simulink model "trajectories"  (R2016b)
settings: Solver=FixedStepAuto  StartTime=0.0  StopTime=20  FixedStep=.1  RelTol=1e-3
undefined symbols (not defined in the file or in its folder): sigbuilder_block
libraries: simulink x3, powerlib_meascontrol x1
settings Model: Creator=Kamran  LastModifiedBy=Kamran

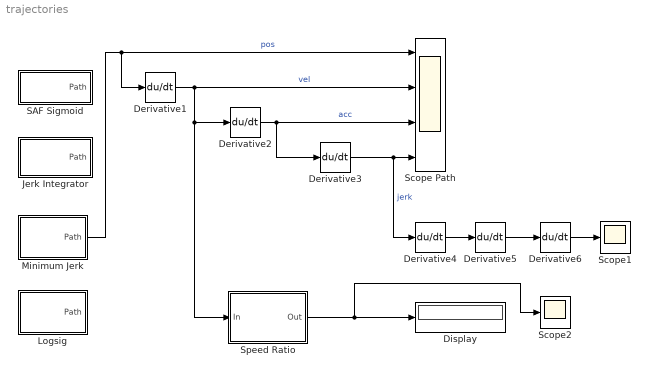
== system trajectories ==
  Derivative{1..6} (6 alike) : Derivative
  Display : Display
  Jerk Integrator : Subsystem
  Logsig : Subsystem
  Minimum Jerk : Subsystem  mask{xi=0, xf=3, d=10, start=5}
      mask prompts: xi "Initial Position"; xf "Final Position"; d "Duration"; start "Start Time"
      mask help: Neville Hogan (1984a) noted that smoothness can be quantified as a function of jerk. This function, among all possible functions, has the minimum jerk cost. Which means that some function that happens to have its sixth derivative equal to zero will minimize your jerk function.
      mask Help: http://www.shadmehrlab.org/book/minimum_jerk/minimumjerk.htm
  SAF Sigmoid : Subsystem
  Scope Path : Scope  NumInputPorts=4
  Scope1 : Scope
  Scope2 : Scope
  Speed Ratio : Subsystem  mask{ts=5, tf=15}
      mask prompts: ts "Measure Start Time"; tf "Measure End Time"
      mask help: Ratio of peak speed to average speed (r). Psychophysical experiments reveal that your reaching movements have a ratio r = 1.75.
      mask Help: http://www.shadmehrlab.org/book/minimum_jerk/minimumjerk.htm
  wires:
  Minimum Jerk/1(Path) -> Scope Path/1, Derivative1/1  "pos"
  Derivative1/1 -> Derivative2/1, Speed Ratio/1(In), Scope Path/2  "vel"
  Derivative3/1 -> Scope Path/4, Derivative4/1  "jerk"
  Derivative2/1 -> Derivative3/1, Scope Path/3  "acc"
  Speed Ratio/1(Out) -> Scope2/1, Display/1
  Derivative5/1 -> Derivative6/1
  Derivative4/1 -> Derivative5/1
  Derivative6/1 -> Scope1/1

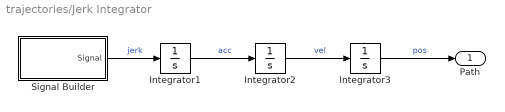
== system trajectories/Jerk Integrator ==
  Integrator1 : Integrator
  Integrator2 : Integrator
  Integrator3 : Integrator
  Signal Builder : Subsystem  Tag=STV Subsys  LoadFcn=sigbuilder_block('load');  StartFcn=sigbuilder_block('start');  StopFcn=sigbuilder_block('stop');  ClipboardFcn=sigbuilder_block('clipboard');  mask(Sigbuilder block){tuvar=[0:10]}
      mask help: Simulink:masks:SigbuilderBlock_MD
      mask init:
      | if ~strcmp(get_param(bdroot(gcbh),'SimulationStatus'),'stopped') tuvar = sigbuilder_block('maskInit'); end
      settings: CopyFcn=sigbuilder_block('copy');  DeleteFcn=sigbuilder_block('delete');  ModelCloseFcn=sigbuilder_block('modelClose');  PreSaveFcn=sigbuilder_block('preSave');  PauseFcn=sigbuilder_block('pause');  ContinueFcn=sigbuilder_block('continue');  NameChangeFcn=sigbuilder_block('namechange');  OpenFcn=sigbuilder_block('open',[6 30 1188 546.75 ]);  CloseFcn=sigbuilder_block('close');
      mask Display: plot(0, 0, 100, 100,[2, 2, 32, 32, 2], [68, 8, 8, 68, 68],[32, 2], [38, 38], [32, 19, 2],[53, 60, 44], [32, 17, 17, 2],[16, 16, 31, 31]);txt = getActiveGroup(gcbh);text(2, 100, txt,'verticalAlignment', 'top');
  Path : Outport
  wires:
  Integrator1/1 -> Integrator2/1  "acc"
  Integrator2/1 -> Integrator3/1  "vel"
  Signal Builder/1(Signal) -> Integrator1/1  "jerk"
  Integrator3/1 -> Path/1  "pos"

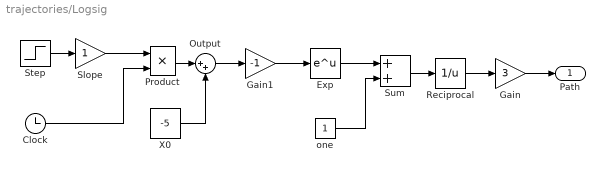
== system trajectories/Logsig ==
  Clock : Clock
      settings: DisableCoverage=on
  Exp : Math  SaturateOnIntegerOverflow=on
  Gain : Gain  Gain=3
  Gain1 : Gain  Gain=-1  SaturateOnIntegerOverflow=on  OutDataTypeStr=Inherit: Same as input  ParamDataTypeStr=Inherit: Same as input
  Output : Sum  Inputs=|++  SaturateOnIntegerOverflow=on  InputSameDT=on  OutDataTypeStr=Inherit: Same as first input
  Product : Product  DisableCoverage=on  SaturateOnIntegerOverflow=on  InputSameDT=on  OutDataTypeStr=Inherit: Same as first input
  Reciprocal : Math  Operator=reciprocal  SaturateOnIntegerOverflow=on
  Slope : Gain
  Step : Step  DisableCoverage=on  Time=0  SampleTime=0
  Sum : Sum  SaturateOnIntegerOverflow=on  InputSameDT=on  OutDataTypeStr=Inherit: Same as first input
  X0 : Constant  Value=-5
  one : Constant
  Path : Outport
  wires:
  Slope/1 -> Product/1
  Step/1 -> Slope/1
  Product/1 -> Output/1
  X0/1 -> Output/2
  Clock/1 -> Product/2
  Sum/1 -> Reciprocal/1
  one/1 -> Sum/2
  Exp/1 -> Sum/1
  Gain1/1 -> Exp/1
  Output/1 -> Gain1/1
  Gain/1 -> Path/1
  Reciprocal/1 -> Gain/1

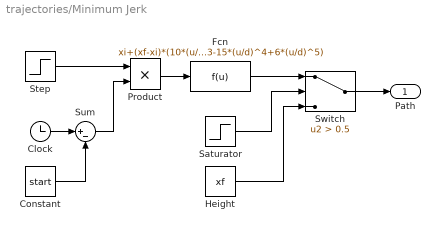
== system trajectories/Minimum Jerk ==
  Clock : Clock
  Constant : Constant  Value=start
  Fcn : Fcn  Expr=xi+(xf-xi)*(10*(u/d)^3-15*(u/d)^4+6*(u/d)^5)
  Height : Constant  Value=xf
  Product : Product
  Saturator : Step  Time=start+d  Before=1  After=0  SampleTime=0
  Step : Step  Time=start  SampleTime=0
  Sum : Sum  Inputs=|+-
  Switch : Switch  Criteria=u2 > Threshold  Threshold=0.5
  Path : Outport
  wires:
  Product/1 -> Fcn/1
  Fcn/1 -> Switch/1
  Step/1 -> Product/1
  Clock/1 -> Sum/1
  Constant/1 -> Sum/2
  Sum/1 -> Product/2
  Saturator/1 -> Switch/2
  Height/1 -> Switch/3
  Switch/1 -> Path/1

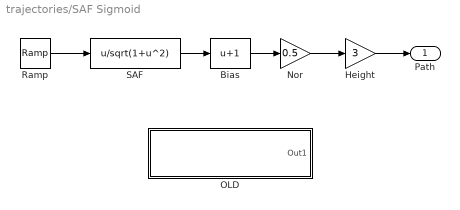
== system trajectories/SAF Sigmoid ==
  Bias : Bias  Bias=1
  Height : Gain  Gain=3
  Nor : Gain  Gain=0.5
  OLD : Subsystem
  Ramp : simulink/Sources/Ramp  slope=1  start=0  X0=-5
  SAF : Fcn  Expr=u/sqrt(1+u^2)
  Path : Outport
  wires:
  Ramp/1 -> SAF/1
  SAF/1 -> Bias/1
  Height/1 -> Path/1
  Bias/1 -> Nor/1
  Nor/1 -> Height/1

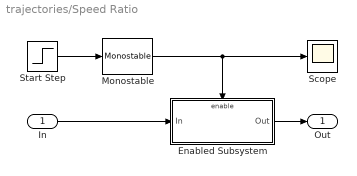
== system trajectories/Speed Ratio ==
  In : Inport
  Enabled Subsystem : Subsystem  TreatAsAtomicUnit=on
  Monostable : powerlib_meascontrol/Logic/Monostable  EdgeDetect=Rising  PulseDuration=tf-ts  ic=0  Ts=0
  Scope : Scope
  Start Step : Step  Time=ts  SampleTime=0
  Out : Outport
  wires:
  In/1 -> Enabled Subsystem/1(In)
  Enabled Subsystem/1(Out) -> Out/1
  Start Step/1 -> Monostable/1
  Monostable/1 -> Scope/1, Enabled Subsystem/Enable

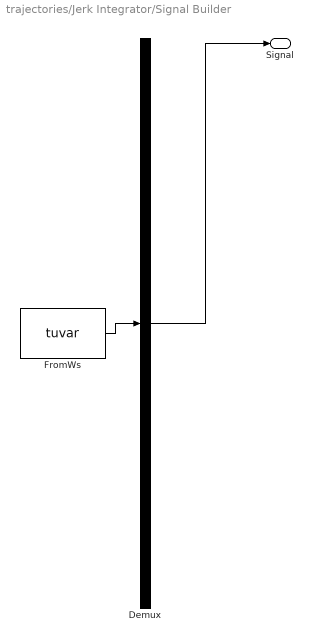
== system trajectories/Jerk Integrator/Signal Builder ==
  Demux : Demux  Tag=STV Demux  Outputs=1
  FromWs : FromWorkspace  Tag=STV FromWs  VariableName=tuvar  SampleTime=0
      SigBuilderData=|
      | common.afterFinalStr = 'Extrapolate'
      | common.sampleTime = 0
      | dataSet.timeRange = [0 10]
      | dataSet.name = 'Group'
      | sbobj.Groups.Name = 'Group'
      | sbobj.Groups.Signals.Name = 'Signal'
      | sbobj.Groups.Signals.XData = [0 1 1 2 2 3 3 4 4 5 5 10]
      | sbobj.Groups.Signals.YData = [1 1 -1 -1 0 0 -1 -1 1 1 0 0]
  Signal : Outport  Tag=STV Outport
  wires:
  Demux/1 -> Signal/1
  FromWs/1 -> Demux/1

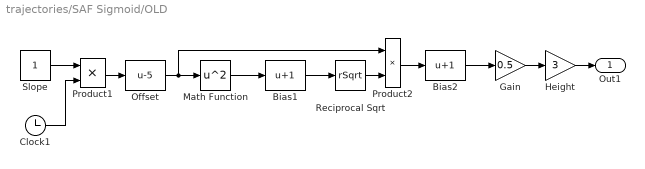
== system trajectories/SAF Sigmoid/OLD ==
  Bias1 : Bias  Bias=1
  Bias2 : Bias  Bias=1
  Clock1 : Clock
      settings: DisableCoverage=on
  Gain : Gain  Gain=0.5
  Height : Gain  Gain=3
  Math Function : Math  Operator=square  SaturateOnIntegerOverflow=on
  Offset : Bias  Bias=-5
  Product1 : Product  DisableCoverage=on  SaturateOnIntegerOverflow=on  InputSameDT=on  OutDataTypeStr=Inherit: Same as first input
  Product2 : Product  DisableCoverage=on  SaturateOnIntegerOverflow=on  InputSameDT=on  OutDataTypeStr=Inherit: Same as first input
  Reciprocal Sqrt : Sqrt  Operator=rSqrt  SaturateOnIntegerOverflow=on
  Slope : Constant
  Out1 : Outport
  wires:
  Bias1/1 -> Reciprocal Sqrt/1
  Reciprocal Sqrt/1 -> Product2/2
  Clock1/1 -> Product1/2
  Slope/1 -> Product1/1
  Product1/1 -> Offset/1
  Math Function/1 -> Bias1/1
  Product2/1 -> Bias2/1
  Offset/1 -> Math Function/1, Product2/1
  Bias2/1 -> Gain/1
  Gain/1 -> Height/1
  Height/1 -> Out1/1

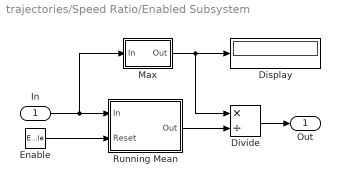
== system trajectories/Speed Ratio/Enabled Subsystem ==
  In : Inport
  Enable : EnablePort  ShowOutputPort=on
  Display : Display
  Divide : Product  Inputs=*/
  Max : Subsystem
  Running Mean : Subsystem
  Out : Outport
  wires:
  In/1 -> Running Mean/1(In), Max/1(In)
  Max/1(Out) -> Display/1, Divide/1
  Running Mean/1(Out) -> Divide/2
  Divide/1 -> Out/1
  Enable/1 -> Running Mean/2(Reset)

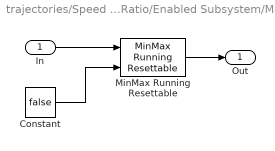
== system trajectories/Speed Ratio/Enabled Subsystem/Max ==
  In : Inport
  Constant : Constant  Value=false
  MinMax Running Resettable : simulink/Math Operations/MinMax Running Resettable  Function=max  vinit=0.0
  Out : Outport
  wires:
  MinMax Running Resettable/1 -> Out/1
  Constant/1 -> MinMax Running Resettable/2
  In/1 -> MinMax Running Resettable/1

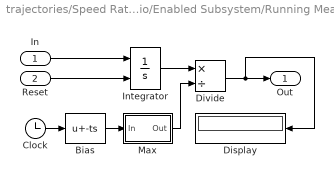
== system trajectories/Speed Ratio/Enabled Subsystem/Running Mean ==
  In : Inport
  Reset : Inport  Port=2
  Bias : Bias  Bias=-ts
  Clock : Clock
  Display : Display
  Divide : Product  Inputs=*/
  Integrator : Integrator  ExternalReset=rising
  Max : Subsystem
  Out : Outport
  wires:
  Clock/1 -> Bias/1
  Integrator/1 -> Divide/1
  In/1 -> Integrator/1
  Max/1(Out) -> Divide/2
  Divide/1 -> Display/1, Out/1
  Reset/1 -> Integrator/2
  Bias/1 -> Max/1(In)

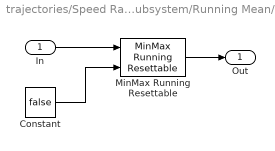
== system trajectories/Speed Ratio/Enabled Subsystem/Running Mean/Max ==
  In : Inport
  Constant : Constant  Value=false
  MinMax Running Resettable : simulink/Math Operations/MinMax Running Resettable  Function=max  vinit=0.0
  Out : Outport
  wires:
  MinMax Running Resettable/1 -> Out/1
  Constant/1 -> MinMax Running Resettable/2
  In/1 -> MinMax Running Resettable/1
